simulink model "Batter_Model_01_1"  (Simulink 8.9)
settings: Solver=ode45  StartTime=0.0  StopTime=10.0  RelTol=1e-3  EnableMultiTasking=on
settings Model: SuppressorTable=22 serialization::archive 11 0 6 0 0 0 0 0  Creator=hlopez5  LastModifiedBy=judithlopez
settings DataIOCC: SignalLoggingSaveFormat=Dataset
settings DebuggingCC: UnderspecifiedInitializationDetection=Simplified  MergeDetectMultiDrivingBlocksExec=error  SolverPrmCheckMsg=warning  FcnCallInpInsideContextMsg=error
settings GRTTargetCC: CombineOutputUpdateFcns=on  GRTInterface=off

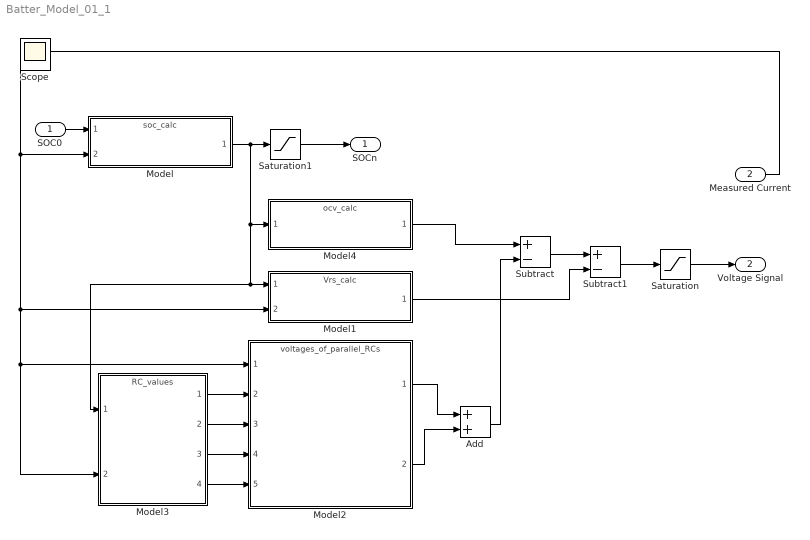
== system Batter_Model_01_1 ==
  SOC0 : Inport
  Measured Current : Inport  Port=2
  Add : Sum
  Model : ModelReference  ModelNameDialog=soc_calc.mdl  SimulationMode=Normal  ModelReferenceVersion=1.3
  Model1 : ModelReference  ModelNameDialog=Vrs_calc.mdl  SimulationMode=Normal  ModelReferenceVersion=1.2
  Model2 : ModelReference  ModelNameDialog=voltages_of_parallel_RCs.mdl  SimulationMode=Normal  ModelReferenceVersion=1.4
  Model3 : ModelReference  ModelNameDialog=RC_values.mdl  SimulationMode=Normal  ModelReferenceVersion=1.5
  Model4 : ModelReference  ModelNameDialog=ocv_calc.mdl  SimulationMode=Normal  ModelReferenceVersion=1.3
  Saturation : Saturate  UpperLimit=12  LowerLimit=1
  Saturation1 : Saturate  UpperLimit=500  LowerLimit=-500
  Subtract : Sum  Inputs=+-
  Subtract1 : Sum  Inputs=+-
  SOCn : Outport
  Voltage Signal : Outport  Port=2
  Scope : Scope
  wires:
  Model3/1 -> Model2/2
  Model3/2 -> Model2/3
  Model3/3 -> Model2/4
  Model3/4 -> Model2/5
  Model2/1 -> Add/1
  Model2/2 -> Add/2
  Model4/1 -> Subtract/1
  Add/1 -> Subtract/2
  Subtract/1 -> Subtract1/1
  Model1/1 -> Subtract1/2
  Subtract1/1 -> Saturation/1
  SOC0/1 -> Model/1
  Model/1 -> Model3/1, Model1/1, Model4/1, Saturation1/1
  Saturation1/1 -> SOCn/1
  Measured Current/1 -> Model3/2, Model2/1, Model1/2, Model/2
  Saturation/1 -> Voltage Signal/1
